simulink model "least_square_2ordem_des"  (Simulink 10.3)
settings: Solver=ode45  StartTime=10  StopTime=20  RelTol=1e-3  AbsTol=1e-6
values from neighbouring files (symbols this model uses):
  As = 2    [sim_grad_norm_2ordem.m]
  DC = 1    [sim_grad_norm_2ordem.m]
  gamma1 = 1*eye(4)    [sim_grad_norm_2ordem.m]
  gamma2 = 0    [sim_grad_norm_2ordem.m]
  kappa = 0    [sim_grad_norm_2ordem.m]
  lambda0 = 1    [sim_grad_norm_2ordem.m]
  lambda1 = 2    [sim_grad_norm_2ordem.m]
  lambda2 = 3    [sim_grad_norm_2ordem.m]
  P01 = 1*eye(4)    [sim_grad_norm_2ordem.m]
  st = 0.01    [sim_grad_norm_2ordem.m]
  theta0 = [0;0;0;0]    [sim_grad_norm_2ordem.m]
  theta_star1 = [b0; b1; a0; a1]    [sim_grad_norm_2ordem.m]
  theta_star2 = theta_star1    [sim_grad_norm_2ordem.m]
  ws = 0.1*pi    (= 0.314159265359)    [sim_grad_norm_2ordem.m]
libraries: cstblocks x1
settings Model: LogicAnalyzerSignalOrdering=70793da9-eb15-4f57-99ee-5707dcc79d9b,2ef5c575-fcfa-49cc-b545-e8a8b41c0ea7,fea41da3-d57e-44aa-96d4-4ceda414349f,b400014a-40bf-49f6-9e38-b7c144e10992,5c3de4f8-109d-4fd1-ba0b-6334d0ea49c7,919e012d-1cd0-4a05-ae56-aa165e610728,b5ac2b2c-b937-4eec-9749-971b2015543d,88bff409-99b8-467d-9ac1-db9407d296a2,8f7b36af-7405-431b-9f2e-81f8b2f0f1ee  Creator=Ramon  LastModifiedBy=linco  MultithreadedSim=on
settings SolverCC: AutoScaleAbsTol=off
settings DataIOCC: SaveOutput=off  SaveTime=off
settings OptimizationCC: BlockReduction=off  BooleanDataType=off  InitFltsAndDblsToZero=on
settings DebuggingCC: SaveWithParameterizedLinksMsg=none  SignalResolutionControl=TryResolveAllWithWarning  MultiTaskDSMMsg=warning  MultiTaskCondExecSysMsg=none
settings HardwareCC: TargetUnknown=on
settings RTWCC: TemplateMakefile=grt_vc.tmf

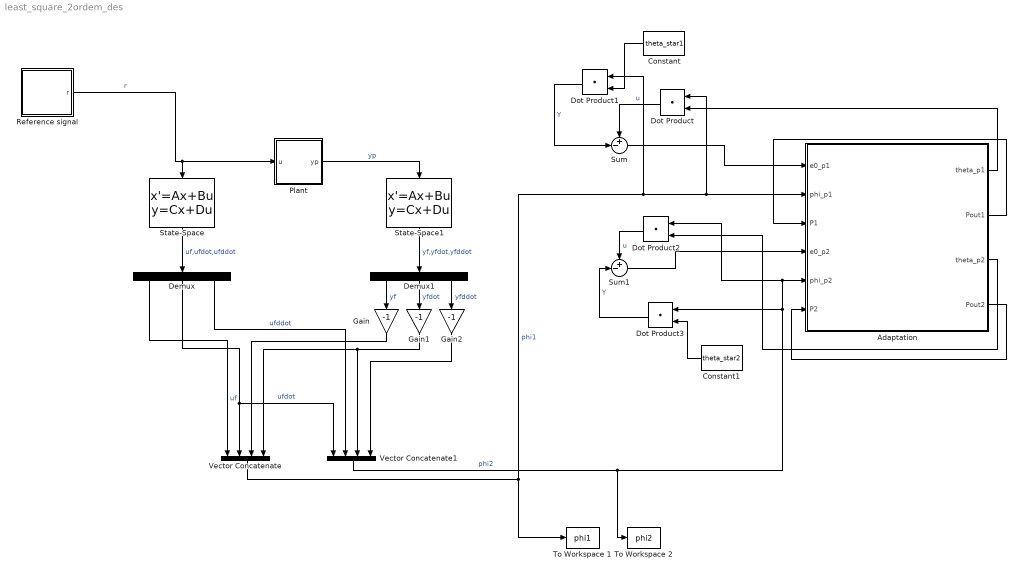
== system least_square_2ordem_des ==
  Adaptation : Subsystem
  Constant : Constant  Value=theta_star1
  Constant1 : Constant  Value=theta_star2
  Demux : Demux  Outputs=3
  Demux1 : Demux  Outputs=3
  Dot Product{,1..3} (4 alike) : DotProduct  InputSameDT=on  OutDataTypeStr=Inherit: Inherit via internal rule
  Gain : Gain  Gain=-1
  Gain1 : Gain  Gain=-1
  Gain2 : Gain  Gain=-1
  Plant : Subsystem
  Reference signal : Subsystem
  State-Space : StateSpace  A=[0 1 0;0 0 1; -lambda0 -lambda1 -lambda2]  B=[0; 0; 1]  C=[1 0 0;0 1 0; 0 0 1]  D=[0;0;0]  InitialCondition=0
  State-Space1 : StateSpace  A=[0 1 0;0 0 1; -lambda0 -lambda1 -lambda2]  B=[0; 0; 1]  C=[1 0 0;0 1 0; 0 0 1]  D=[0;0;0]  InitialCondition=0
  Sum : Sum  Inputs=+-|
  Sum1 : Sum  Inputs=+-|
  To Workspace 1 : ToWorkspace  VariableName=phi1  SampleTime=st
  To Workspace 2 : ToWorkspace  VariableName=phi2  SampleTime=st
  Vector Concatenate : Concatenate  NumInputs=4
  Vector Concatenate1 : Concatenate  NumInputs=4
  wires:
  Adaptation/1(theta_p1) -> Dot Product/2
  Reference signal/1(r) -> State-Space/1, Plant/1(u)  "r"
  Plant/1(yp) -> State-Space1/1  "yp"
  Sum/1 -> Adaptation/1(e0_p1)
  Dot Product/1 -> Sum/1  "u"
  Constant/1 -> Dot Product1/2
  Dot Product1/1 -> Sum/2  "Y"
  Adaptation/2(Pout1) -> Adaptation/3(P1)
  Adaptation/4(Pout2) -> Adaptation/6(P2)
  State-Space/1 -> Demux/1  "uf,ufdot,ufddot"
  State-Space1/1 -> Demux1/1  "yf,yfdot,yfddot"
  Demux/1 -> Vector Concatenate/1  "uf"
  Demux/2 -> Vector Concatenate1/1, Vector Concatenate/2  "ufdot"
  Demux/3 -> Vector Concatenate1/2  "ufddot"
  Demux1/1 -> Gain/1  "yf"
  Demux1/2 -> Gain1/1  "yfdot"
  Demux1/3 -> Gain2/1  "yfddot"
  Gain/1 -> Vector Concatenate/3
  Gain1/1 -> Vector Concatenate1/3, Vector Concatenate/4
  Vector Concatenate/1 -> To Workspace 1/1, Dot Product1/1, Dot Product/1, Adaptation/2(phi_p1)  "phi1"
  Vector Concatenate1/1 -> To Workspace 2/1, Dot Product3/1, Dot Product2/1, Adaptation/5(phi_p2)  "phi2"
  Gain2/1 -> Vector Concatenate1/4
  Sum1/1 -> Adaptation/4(e0_p2)
  Constant1/1 -> Dot Product3/2
  Dot Product3/1 -> Sum1/2  "Y"
  Adaptation/3(theta_p2) -> Dot Product2/2
  Dot Product2/1 -> Sum1/1  "u"

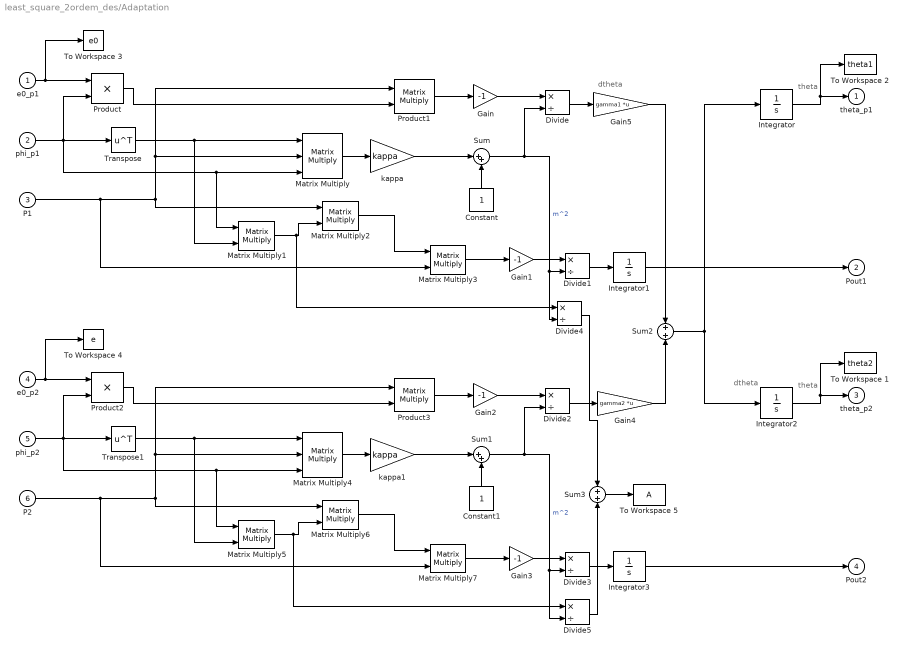
== system least_square_2ordem_des/Adaptation ==
  note: theta
  note: dtheta
  note: theta
  note: dtheta
  e0_p1 : Inport  PortDimensions=1
  phi_p1 : Inport  Port=2
  P1 : Inport  Port=3
  e0_p2 : Inport  Port=4  PortDimensions=1
  phi_p2 : Inport  Port=5
  P2 : Inport  Port=6
  Constant : Constant
  Constant1 : Constant
  Divide{,1..5} (6 alike) : Product  Inputs=*/
  Gain{,1..3} (4 alike) : Gain  Gain=-1
  Gain4 : Gain  Gain=gamma2  Multiplication=Matrix(K*u)
  Gain5 : Gain  Gain=gamma1  Multiplication=Matrix(K*u)
  Integrator : Integrator  InitialCondition=theta0
  Integrator1 : Integrator  InitialCondition=P01
  Integrator2 : Integrator  InitialCondition=theta0
  Integrator3 : Integrator  InitialCondition=P01
  Matrix Multiply : Product  Inputs=3  Multiplication=Matrix(*)
  Matrix Multiply{1..3,5..7} (6 alike) : Product  Multiplication=Matrix(*)
  Matrix Multiply4 : Product  Inputs=3  Multiplication=Matrix(*)
  Product : Product  InputSameDT=on  RndMeth=Zero  SaturateOnIntegerOverflow=on  OutDataTypeStr=Inherit: Same as first input
  Product1 : Product  Multiplication=Matrix(*)
  Product2 : Product  InputSameDT=on  RndMeth=Zero  SaturateOnIntegerOverflow=on  OutDataTypeStr=Inherit: Same as first input
  Product3 : Product  Multiplication=Matrix(*)
  Sum : Sum  Inputs=|++
  Sum1 : Sum  Inputs=|++
  Sum2 : Sum
  Sum3 : Sum
  To Workspace 1 : ToWorkspace  VariableName=theta2  SampleTime=st
  To Workspace 2 : ToWorkspace  VariableName=theta1  SampleTime=st
  To Workspace 3 : ToWorkspace  VariableName=e0  SampleTime=st
  To Workspace 4 : ToWorkspace  VariableName=e  SampleTime=st
  To Workspace 5 : ToWorkspace  VariableName=A  SampleTime=st
  Transpose : Math  Operator=transpose  SaturateOnIntegerOverflow=on
  Transpose1 : Math  Operator=transpose  SaturateOnIntegerOverflow=on
  kappa : Gain  Gain=kappa  SaturateOnIntegerOverflow=on  OutDataTypeStr=Inherit: Same as input  ParamDataTypeStr=Inherit: Same as input
  kappa1 : Gain  Gain=kappa  SaturateOnIntegerOverflow=on  OutDataTypeStr=Inherit: Same as input  ParamDataTypeStr=Inherit: Same as input
  theta_p1 : Outport  InitialOutput=0  VectorParamsAs1DForOutWhenUnconnected=off
  Pout1 : Outport  Port=2  InitialOutput=0  VectorParamsAs1DForOutWhenUnconnected=off
  theta_p2 : Outport  Port=3  InitialOutput=0  VectorParamsAs1DForOutWhenUnconnected=off
  Pout2 : Outport  Port=4  InitialOutput=0  VectorParamsAs1DForOutWhenUnconnected=off
  wires:
  Integrator/1 -> To Workspace 2/1, theta_p1/1
  Gain5/1 -> Sum2/1
  phi_p1/1 -> Transpose/1, Matrix Multiply1/1, Matrix Multiply/3, Product/2
  e0_p1/1 -> Product/1, To Workspace 3/1
  Product1/1 -> Gain/1
  Product/1 -> Product1/2
  Matrix Multiply/1 -> kappa/1
  Constant/1 -> Sum/2
  kappa/1 -> Sum/1
  Sum/1 -> Divide4/2, Divide1/2, Divide/2  "m^2"
  Integrator1/1 -> Pout1/1
  P1/1 -> Matrix Multiply3/2, Matrix Multiply2/1, Matrix Multiply/2, Product1/1
  Gain/1 -> Divide/1
  Divide1/1 -> Integrator1/1
  Transpose/1 -> Matrix Multiply1/2, Matrix Multiply/1
  Matrix Multiply1/1 -> Divide4/1, Matrix Multiply2/2
  Matrix Multiply2/1 -> Matrix Multiply3/1
  Matrix Multiply3/1 -> Gain1/1
  Gain1/1 -> Divide1/1
  Matrix Multiply4/1 -> kappa1/1
  Gain3/1 -> Divide3/1
  Matrix Multiply7/1 -> Gain3/1
  Matrix Multiply6/1 -> Matrix Multiply7/1
  P2/1 -> Matrix Multiply7/2, Matrix Multiply6/1, Matrix Multiply4/2, Product3/1
  Matrix Multiply5/1 -> Divide5/1, Matrix Multiply6/2
  Constant1/1 -> Sum1/2
  Transpose1/1 -> Matrix Multiply5/2, Matrix Multiply4/1
  Divide3/1 -> Integrator3/1
  Sum1/1 -> Divide5/2, Divide3/2, Divide2/2  "m^2"
  Integrator3/1 -> Pout2/1
  Product3/1 -> Gain2/1
  kappa1/1 -> Sum1/1
  Product2/1 -> Product3/2
  e0_p2/1 -> Product2/1, To Workspace 4/1
  Gain2/1 -> Divide2/1
  Divide2/1 -> Gain4/1
  Integrator2/1 -> To Workspace 1/1, theta_p2/1
  phi_p2/1 -> Transpose1/1, Matrix Multiply5/1, Matrix Multiply4/3, Product2/2
  Sum2/1 -> Integrator/1, Integrator2/1
  Gain4/1 -> Sum2/2
  Divide/1 -> Gain5/1
  Sum3/1 -> To Workspace 5/1
  Divide4/1 -> Sum3/1
  Divide5/1 -> Sum3/2

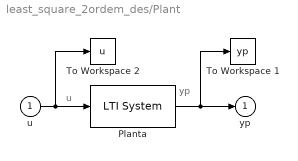
== system least_square_2ordem_des/Plant ==
  note: yp
  note: u
  u : Inport
  Planta : cstblocks/LTI System  sys=P  IC=x0
  To Workspace 1 : ToWorkspace  VariableName=yp  SampleTime=st
  To Workspace 2 : ToWorkspace  VariableName=u  SampleTime=st
  yp : Outport  InitialOutput=0  VectorParamsAs1DForOutWhenUnconnected=off
  wires:
  u/1 -> To Workspace 2/1, Planta/1
  Planta/1 -> yp/1, To Workspace 1/1

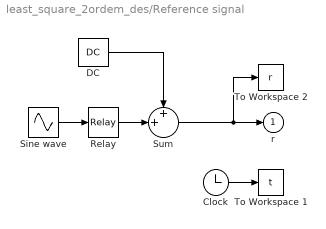
== system least_square_2ordem_des/Reference signal ==
  Clock : Clock
  DC : Constant  Value=DC
  Relay : Relay  OnOutputValue=As  OffOutputValue=-As
  Sine wave : Sin  Frequency=ws  SampleTime=0
  Sum : Sum  Inputs=++|  InputSameDT=on  SaturateOnIntegerOverflow=on  OutDataTypeStr=Inherit: Same as first input
  To Workspace 1 : ToWorkspace  VariableName=t  SampleTime=st
  To Workspace 2 : ToWorkspace  VariableName=r  SampleTime=st
  r : Outport  InitialOutput=0  VectorParamsAs1DForOutWhenUnconnected=off
  wires:
  DC/1 -> Sum/1
  Sum/1 -> r/1, To Workspace 2/1
  Clock/1 -> To Workspace 1/1
  Sine wave/1 -> Relay/1
  Relay/1 -> Sum/2
